simulink library "proplsn_lib"  (R2018b)
settings: Solver=VariableStepAuto  StartTime=0.0  StopTime=10.0  RelTol=1e-3
undefined symbols (not defined in the file or in its folder): battery_bkpt_chg_st_dec, proplsn, simm
libraries: $bdroot x1
settings Model: Creator=Kevin  LastModifiedBy=austi
settings SFSimCC: SimUseLocalCustomCode=off
settings RTWCC: RTWUseLocalCustomCode=off
settings CodeAppCC: StateflowObjectComments=on

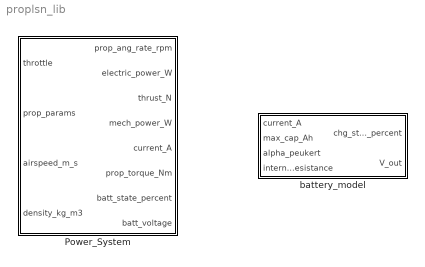
== system proplsn_lib ==
  Power_System : Subsystem
  battery_model : Subsystem

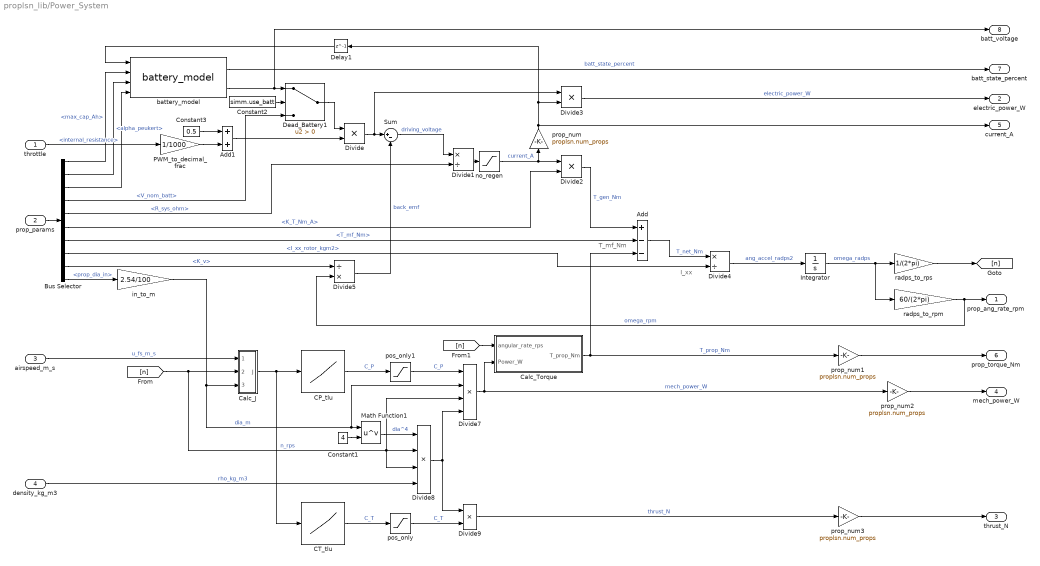
== system proplsn_lib/Power_System ==
  note: I_xx
  note: T_mf_Nm
  throttle : Inport
  prop_params : Inport  Port=2
  airspeed_m_s : Inport  Port=3
  density_kg_m3 : Inport  Port=4
  Add : Sum  Inputs=+--
  Add1 : Sum
  Bus Selector : BusSelector  OutputSignals=max_cap_Ah,alpha_peukert,internal_resistance,V_nom_batt,R_sys_ohm,K_T_Nm_A,T_mf_Nm,I_xx_rotor_kgm2,K_v,prop_dia_in
  CP_tlu : Lookup_n-D  NumberOfTableDimensions=1  BreakpointsForDimension1=proplsn.CP_bkpt  Table=proplsn.CP_tlu  InternalRulePriority=Speed  RndMeth=Simplest  InputSameDT=on
  CT_tlu : Lookup_n-D  NumberOfTableDimensions=1  BreakpointsForDimension1=proplsn.CT_bkpt  Table=proplsn.CT_tlu  InternalRulePriority=Speed  RndMeth=Simplest  InputSameDT=on
  Calc_J : Subsystem
  Calc_Torque : Subsystem
  Constant1 : Constant  Value=4
  Constant2 : Constant  Value=simm.use_batt  OutDataTypeStr=boolean
  Constant3 : Constant  Value=0.5
  Dead_Battery1 : Switch  Criteria=u2 > Threshold
  Delay1 : Delay  DelayLength=1
  Divide{,2..3,9} (4 alike) : Product  Inputs=**
  Divide1 : Product  Inputs=*/
  Divide4 : Product  Inputs=*/
  Divide5 : Product  Inputs=/*
  Divide7 : Product  Inputs=****
  Divide8 : Product  Inputs=****
  Integrator : Integrator  InitialCondition=simm.init_omega_radps  LimitOutput=on  LowerSaturationLimit=0
  Math Function1 : Math  Operator=pow  SaturateOnIntegerOverflow=on
  PWM_to_decimal_frac : Gain  Gain=1/1000
  Sum : Sum  Inputs=|+-
  battery_model : $bdroot/battery_model  SystemSampleTime=-1
  in_to_m : Gain  Gain=2.54/100
  no_regen : Saturate  UpperLimit=inf  LowerLimit=0
  pos_only : Saturate  UpperLimit=inf  LowerLimit=0
  pos_only1 : Saturate  UpperLimit=inf  LowerLimit=0
  prop_num{,1..3} (4 alike) : Gain  Gain=proplsn.num_props
  radps_to_rpm : Gain  Gain=60/(2*pi)
  radps_to_rps : Gain  Gain=1/(2*pi)
  prop_ang_rate_rpm : Outport
  electric_power_W : Outport  Port=2
  thrust_N : Outport  Port=3
  mech_power_W : Outport  Port=4
  current_A : Outport  Port=5
  prop_torque_Nm : Outport  Port=6
  batt_state_percent : Outport  Port=7
  batt_voltage : Outport  Port=8
  wires:
  Dead_Battery1/1 -> Divide/1
  Constant2/1 -> Dead_Battery1/2
  battery_model/1 -> batt_state_percent/1  "batt_state_percent"
  Bus Selector/1 -> battery_model/2  "<max_cap_Ah>"
  battery_model/2 -> Dead_Battery1/1, batt_voltage/1
  Bus Selector/10 -> in_to_m/1  "<prop_dia_in>"
  Divide5/1 -> Sum/2  "back_emf"
  radps_to_rpm/1 -> Divide5/2, prop_ang_rate_rpm/1  "omega_rpm"
  Bus Selector/9 -> Divide5/1  "<K_v>"
  Integrator/1 -> radps_to_rps/1, radps_to_rpm/1  "omega_radps"
  Divide4/1 -> Integrator/1  "ang_accel_radps2"
  Bus Selector/8 -> Divide4/2  "<I_xx_rotor_kgm2>"
  Add/1 -> Divide4/1  "T_net_Nm"
  Bus Selector/7 -> Add/2  "<T_mf_Nm>"
  Divide2/1 -> Add/1  "T_gen_Nm"
  Bus Selector/6 -> Divide2/2  "<K_T_Nm_A>"
  Divide3/1 -> electric_power_W/1  "electric_power_W"
  Divide1/1 -> no_regen/1
  Bus Selector/5 -> Divide1/2  "<R_sys_ohm>"
  Sum/1 -> Divide1/1  "driving_voltage"
  Bus Selector/4 -> Dead_Battery1/3  "<V_nom_batt>"
  PWM_to_decimal_frac/1 -> Add1/2
  throttle/1 -> PWM_to_decimal_frac/1
  prop_params/1 -> Bus Selector/1
  radps_to_rps/1 -> [n]
  [n] -> Calc_J/2(n), Divide7/3, Divide8/2, Divide8/3  "n_rps"
  CP_tlu/1 -> pos_only1/1  "C_P"
  Divide7/1 -> prop_num2/1, Calc_Torque/2(Power_W)  "mech_power_W"
  Constant1/1 -> Math Function1/2
  Math Function1/1 -> Divide8/1  "dia^4"
  density_kg_m3/1 -> Divide8/4  "rho_kg_m3"
  CT_tlu/1 -> pos_only/1  "C_T"
  Divide9/1 -> prop_num3/1  "thrust_N"
  Divide8/1 -> Divide7/4, Divide9/1
  in_to_m/1 -> Calc_J/3(D), Divide7/2, Math Function1/1  "dia_m"
  Delay1/1 -> battery_model/1
  Calc_J/1(J) -> CP_tlu/1, CT_tlu/1
  airspeed_m_s/1 -> Calc_J/1(V)  "u_fs_m_s"
  Calc_Torque/1(T_prop_Nm) -> Add/3, prop_num1/1  "T_prop_Nm"
  [n] -> Calc_Torque/1(angular_rate_rps)
  pos_only/1 -> Divide9/2  "C_T"
  pos_only1/1 -> Divide7/1  "C_P"
  Divide/1 -> Divide3/1, Sum/1
  no_regen/1 -> prop_num/1, Divide2/1  "current_A"
  Bus Selector/2 -> battery_model/3  "<alpha_peukert>"
  Bus Selector/3 -> battery_model/4  "<internal_resistance>"
  Add1/1 -> Divide/2
  Constant3/1 -> Add1/1
  prop_num/1 -> Delay1/1, Divide3/2, current_A/1
  prop_num1/1 -> prop_torque_Nm/1
  prop_num2/1 -> mech_power_W/1
  prop_num3/1 -> thrust_N/1

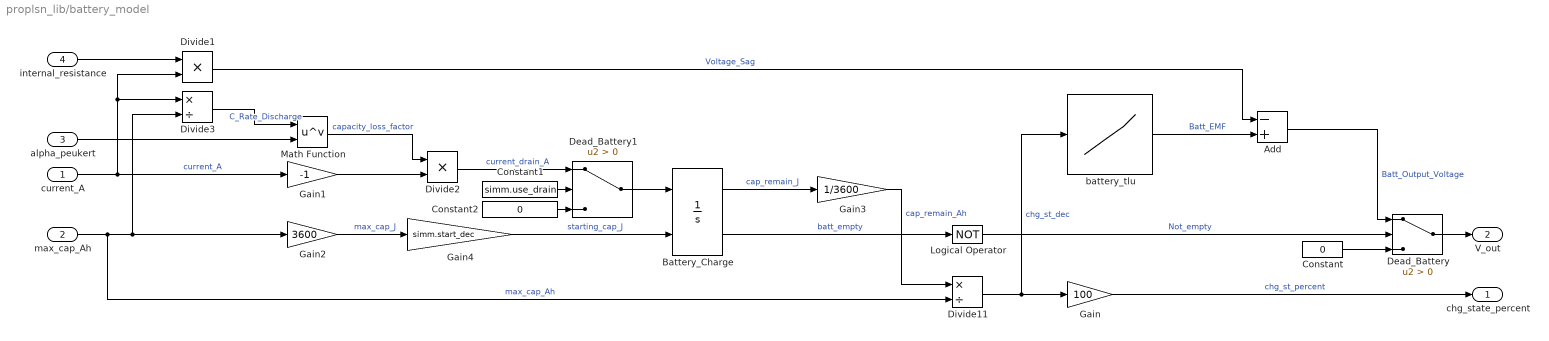
== system proplsn_lib/battery_model ==
  current_A : Inport
  max_cap_Ah : Inport  Port=2
  alpha_peukert : Inport  Port=3
  internal_resistance : Inport  Port=4
  Add : Sum  Inputs=-+
  Battery_Charge : Integrator  InitialConditionSource=external  LimitOutput=on  LowerSaturationLimit=0  ShowSaturationPort=on  ContinuousStateAttributes='cap_remaining'
  Constant : Constant  Value=0
  Constant1 : Constant  Value=simm.use_drain  OutDataTypeStr=boolean
  Constant2 : Constant  Value=0
  Dead_Battery : Switch  Criteria=u2 > Threshold
  Dead_Battery1 : Switch  Criteria=u2 > Threshold
  Divide1 : Product  Inputs=**
  Divide11 : Product  Inputs=*/
  Divide2 : Product  Inputs=**
  Divide3 : Product  Inputs=*/
  Gain : Gain  Gain=100
  Gain1 : Gain  Gain=-1
  Gain2 : Gain  Gain=3600
  Gain3 : Gain  Gain=1/3600
  Gain4 : Gain  Gain=simm.start_dec
  Logical Operator : Logic  Operator=NOT  AllPortsSameDT=off  OutDataTypeStr=boolean
  Math Function : Math  Operator=pow  SaturateOnIntegerOverflow=on
  battery_tlu : Lookup_n-D  NumberOfTableDimensions=1  BreakpointsForDimension1=proplsn.battery_bkpt_chg_st_dec  BreakpointsForDimension2=battery_bkpt_chg_st_dec  Table=proplsn.battery_tlu  ExtrapMethod=Clip  InternalRulePriority=Speed  RndMeth=Simplest  InputSameDT=on
  chg_state_percent : Outport
  V_out : Outport  Port=2
  wires:
  Divide3/1 -> Math Function/1  "C_Rate_Discharge"
  Math Function/1 -> Divide2/1  "capacity_loss_factor"
  alpha_peukert/1 -> Math Function/2
  Gain1/1 -> Divide2/2
  Dead_Battery1/1 -> Battery_Charge/1
  Constant2/1 -> Dead_Battery1/3
  Constant1/1 -> Dead_Battery1/2
  Gain4/1 -> Battery_Charge/2  "starting_cap_J"
  max_cap_Ah/1 -> Gain2/1, Divide3/2, Divide11/2  "max_cap_Ah"
  current_A/1 -> Divide3/1, Divide1/2, Gain1/1  "current_A"
  Divide2/1 -> Dead_Battery1/1  "current_drain_A"
  Gain2/1 -> Gain4/1  "max_cap_J"
  Battery_Charge/1 -> Gain3/1  "cap_remain_J"
  Gain3/1 -> Divide11/1  "cap_remain_Ah"
  Divide11/1 -> battery_tlu/1, Gain/1  "chg_st_dec"
  Gain/1 -> chg_state_percent/1  "chg_st_percent"
  Dead_Battery/1 -> V_out/1
  Constant/1 -> Dead_Battery/3
  Battery_Charge/2 -> Logical Operator/1  "batt_empty"
  Logical Operator/1 -> Dead_Battery/2  "Not_empty"
  battery_tlu/1 -> Add/2  "Batt_EMF"
  internal_resistance/1 -> Divide1/1
  Divide1/1 -> Add/1  "Voltage_Sag"
  Add/1 -> Dead_Battery/1  "Batt_Output_Voltage"

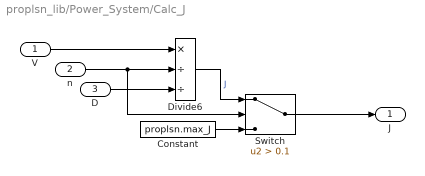
== system proplsn_lib/Power_System/Calc_J ==
  V : Inport
  n : Inport  Port=2
  D : Inport  Port=3
  Constant : Constant  Value=proplsn.max_J
  Divide6 : Product  Inputs=*//
  Switch : Switch  Criteria=u2 > Threshold  Threshold=0.1
  J : Outport
  wires:
  Divide6/1 -> Switch/1  "J"
  V/1 -> Divide6/1
  D/1 -> Divide6/3
  n/1 -> Switch/2, Divide6/2
  Switch/1 -> J/1
  Constant/1 -> Switch/3

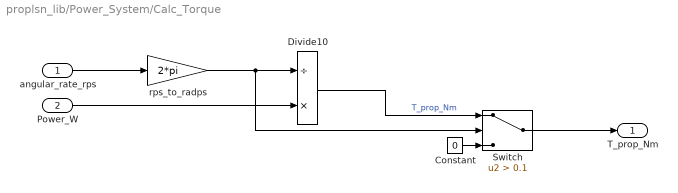
== system proplsn_lib/Power_System/Calc_Torque ==
  angular_rate_rps : Inport
  Power_W : Inport  Port=2
  Constant : Constant  Value=0
  Divide10 : Product  Inputs=/*
  Switch : Switch  Criteria=u2 > Threshold  Threshold=0.1
  rps_to_radps : Gain  Gain=2*pi
  T_prop_Nm : Outport
  wires:
  Divide10/1 -> Switch/1  "T_prop_Nm"
  Power_W/1 -> Divide10/2
  Constant/1 -> Switch/3
  rps_to_radps/1 -> Switch/2, Divide10/1
  Switch/1 -> T_prop_Nm/1
  angular_rate_rps/1 -> rps_to_radps/1
